simulink model "local_sequencer_harness1"  (R2018b)
settings: Solver=FixedStepDiscrete  StartTime=0  StopTime=8  FixedStep=1  RelTol=1e-3
undefined symbols (not defined in the file or in its folder): eof, sigbuilder_block, sldvsubsys, StateFlowModeType
libraries: sldvlib x21, simulink x6, hdlsllib x4
(part 2 of 2)

== stateflow chart local_sequencer_harness1/Test Unit (copied from local_sequencer)/Local Sequencer Subsystem/StateFlow ==
  settings: stateMachineType=MOORE_MACHINE  initializeOutput=1
  note: Make trigger and enable to chart?
  state INIT
    task_done = false;
    task_error = false;
    write = false;
    load_counter = false;
    ctrl = false;
    abort = false;
    increment = false;
    latch_inst_start = false;
    latch_addr = false;
    latch_function = false;
    reset = true;
  state FB_SELECT
    state LOAD_INST_START
      task_done = false;
      task_error = false;
      write = false;
      ctrl = false;
      abort = false;
      load_counter = true;
      increment = false;
      latch_inst_start = false;
      latch_addr = false;
      latch_function = false;
      reset = false;
    state LATCH_INST_START
      task_done = false;
      task_error = false;
      write = false;
      ctrl = false;
      abort = false;
      load_counter = false;
      increment = false;
      latch_inst_start = true;
      latch_addr = false;
      latch_function = true;
      reset = false;
    state INCREMENT_INST
      task_done = false;
      task_error = false;
      write = false;
      ctrl = false;
      abort = false;
      load_counter = false;
      increment = true;
      latch_inst_start = false;
      latch_addr = false;
      latch_function = false;
      reset = false;
    state INST_WAIT
      task_done = false;
      task_error = false;
      write = false;
      ctrl = false;
      abort = false;
      load_counter = false;
      increment = false;
      latch_inst_start = false;
      latch_addr = false;
      latch_function = false;
      reset = false;
    (default) -> LOAD_INST_START [order 1] : [recoverable]
    (default) -> LATCH_INST_START [order 2]
    LATCH_INST_START -> (junction 371)
    LOAD_INST_START -> (junction 371)
    (junction 371) -> FB_SELECT.INCREMENT_INST
    FB_SELECT.INCREMENT_INST -> FB_SELECT.INST_WAIT
  state FETCH
    state CTRL_LO
      task_done = false;
      task_error = false;
      write = false;
      ctrl = false;
      abort = false;
      load_counter = false;
      increment = false;
      latch_inst_start = false;
      latch_addr = false;
      latch_function = false;
      reset = false;
    state INCREMENT_INST
      task_done = false;
      task_error = false;
      write = false;
      ctrl = false;
      abort = false;
      load_counter = false;
      increment = true;
      latch_inst_start = false;
      latch_addr = false;
      latch_function = false;
      reset = false;
    state CTRL_HI
      task_done = false;
      task_error = false;
      write = false;
      ctrl = true;
      abort = false;
      load_counter = false;
      increment = false;
      latch_inst_start = false;
      latch_addr = false;
      latch_function = false;
      reset = false;
    state INST_WAIT
      task_done = false;
      task_error = false;
      write = false;
      ctrl = false;
      abort = false;
      load_counter = false;
      increment = false;
      latch_inst_start = false;
      latch_addr = false;
      latch_function = false;
      reset = false;
    state LATCH_ADDR
      task_done = false;
      task_error = false;
      write = false;
      ctrl = false;
      abort = false;
      load_counter = false;
      increment = false;
      latch_inst_start = false;
      latch_addr = true;
      latch_function = false;
      reset = false;
    state MEM_WAIT
      task_done = false;
      task_error = false;
      write = false;
      ctrl = false;
      abort = false;
      load_counter = false;
      increment = false;
      latch_inst_start = false;
      latch_addr = false;
      latch_function = false;
      reset = false;
    (default) -> FETCH.LATCH_ADDR
    FETCH.CTRL_LO -> FETCH.INCREMENT_INST
    FETCH.CTRL_HI -> FETCH.CTRL_LO
    FETCH.LATCH_ADDR -> MEM_WAIT
    MEM_WAIT -> FETCH.CTRL_HI
    FETCH.INCREMENT_INST -> FETCH.INST_WAIT
  state FB_EXECUTE
    state CTRL_HI
      task_done = false;
      task_error = false;
      write = false;
      ctrl = true;
      abort = false;
      load_counter = false;
      increment = false;
      latch_inst_start = false;
      latch_addr = false;
      latch_function = false;
      reset = false;
    state CTRL_LO
      task_done = false;
      task_error = false;
      write = false;
      ctrl = false;
      abort = false;
      load_counter = false;
      increment = false;
      latch_inst_start = false;
      latch_addr = false;
      latch_function = false;
      reset = false;
    (default) -> FB_EXECUTE.CTRL_HI
    FB_EXECUTE.CTRL_HI -> FB_EXECUTE.CTRL_LO
  state ERROR_STATE
    state CTRL_HI
      %set control and clear init
      task_done = false;
      task_error = false;
      write = false;
      ctrl = true;
      abort = false;
      load_counter = false;
      increment = false;
      latch_inst_start = false;
      latch_addr = false;
      latch_function = false;
      reset = false;
    state ABORT_CTRL_LO
      %task_error and init
      %unchanged
      task_done = false;
      task_error = task_error;
      write = false;
      ctrl = false;
      abort = false;
      load_counter = false;
      increment = false;
      latch_inst_start = false;
      latch_addr = false;
      latch_function = false;
      reset = false;
    state ABORT_CTRL_HI
      %set control, abort, and init
      task_done = false;
      task_error = true;
      write = false;
      ctrl = true;
      abort = true;
      load_counter = false;
      increment = false;
      latch_inst_start = false;
      latch_addr = false;
      latch_function = false;
      reset = false;
    (default) -> ERROR_STATE.CTRL_HI [order 1] : [recoverable]
    ERROR_STATE.CTRL_HI -> (junction 308)
    (default) -> ABORT_CTRL_HI [order 2]
    (junction 308) -> ABORT_CTRL_LO
    ABORT_CTRL_HI -> (junction 308)
  state WRITE
    state WRITE
      task_done = false;
      task_error = false;
      write = true;
      ctrl = false;
      abort = false;
      load_counter = false;
      increment = false;
      latch_inst_start = false;
      latch_addr = false;
      latch_function = false;
      reset = false;
    state INCREMENT_INST
      task_done = false;
      task_error = false;
      write = false;
      ctrl = false;
      abort = false;
      load_counter = false;
      increment = true;
      latch_inst_start = false;
      latch_addr = false;
      latch_function = false;
      reset = false;
    state CTRL_LO
      task_done = false;
      task_error = false;
      write = false;
      ctrl = false;
      abort = false;
      load_counter = false;
      increment = false;
      latch_inst_start = false;
      latch_addr = false;
      latch_function = false;
      reset = false;
    state CTRL_HI
      task_done = false;
      task_error = false;
      write = false;
      ctrl = true;
      abort = false;
      load_counter = false;
      increment = false;
      latch_inst_start = false;
      latch_addr = false;
      latch_function = false;
      reset = false;
    state LATCH_ADDR
      %latch current address
      task_done = false;
      task_error = false;
      write = false;
      ctrl = false;
      abort = false;
      load_counter = false;
      increment = false;
      latch_inst_start = false;
      latch_addr = true;
      latch_function = false;
      reset = false;
    state INST_WAIT
      task_done = false;
      task_error = false;
      write = false;
      ctrl = false;
      abort = false;
      load_counter = false;
      increment = false;
      latch_inst_start = false;
      latch_addr = false;
      latch_function = false;
      reset = false;
    (default) -> WRITE.LATCH_ADDR
    WRITE.LATCH_ADDR -> WRITE.CTRL_HI
    WRITE.CTRL_HI -> WRITE.CTRL_LO
    WRITE.WRITE -> WRITE.INCREMENT_INST
    WRITE.CTRL_LO -> WRITE.WRITE
    WRITE.INCREMENT_INST -> WRITE.INST_WAIT
  state FB_DONE
    state CTRL_HI
      task_done = false;
      task_error = false;
      write = false;
      ctrl = true;
      abort = false;
      load_counter = false;
      increment = false;
      latch_inst_start = false;
      latch_addr = false;
      latch_function = false;
      reset = false;
    state CTRL_LO
      task_done = false;
      task_error = false;
      write = false;
      ctrl = false;
      abort = false;
      load_counter = false;
      increment = false;
      latch_inst_start = false;
      latch_addr = false;
      latch_function = false;
      reset = false;
    (default) -> FB_DONE.CTRL_HI
    FB_DONE.CTRL_HI -> FB_DONE.CTRL_LO
  state TASK_DONE
    %signal task done
    task_done = true;
    task_error = false;
    write = false;
    ctrl = false;
    abort = false;
    load_counter = false;
    increment = false;
    latch_inst_start = false;
    latch_addr = false;
    latch_function = false;
    reset = false;
  FB_SELECT.INST_WAIT -> FETCH
  WRITE.INST_WAIT -> (junction 207)
  FB_DONE.CTRL_LO -> (junction 315) : [new_state]
  FB_EXECUTE.CTRL_LO -> WRITE : [new_state]
  FETCH.INST_WAIT -> (junction 204)
  ABORT_CTRL_LO -> (junction 220)
  (default) -> INIT
  (junction 220) -> INIT [order 2] : [~trigger]
  TASK_DONE -> INIT : [~trigger]
  INIT -> FB_SELECT : [trigger]
  (junction 220) -> FB_SELECT [order 1] : [recoverable]
  (junction 315) -> FB_SELECT [order 2]
  FETCH -> (junction 197)
  (junction 204) -> FETCH [order 2] : [state_iteration]
  (junction 204) -> FB_EXECUTE [order 1] : [new_state]
  FB_EXECUTE -> (junction 197)
  (junction 197) -> ERROR_STATE : [error]
  WRITE -> (junction 197)
  (junction 207) -> WRITE [order 2] : [state_iteration]
  (junction 207) -> FB_DONE [order 1] : [new_state]
  (junction 315) -> TASK_DONE [order 1] : [eof]
  data: task_done output boolean; task_error output boolean; write output boolean; ctrl output boolean; abort output boolean; load_counter output boolean; increment output boolean; latch_inst_start output boolean; latch_addr output boolean; latch_function output boolean; trigger input boolean; error input boolean; state_iteration input boolean; reset output boolean; new_state input boolean; recoverable input boolean; eof input boolean; StateFlowModeLS output Enum: StateFlowModeType

== matlab function local_sequencer_harness1/Test Unit (copied from local_sequencer)/Local Sequencer Subsystem/MATLAB Function ==
  data: code input; y output
function y = recoverable(code)
%#codegen

if(code)
    y = true;
else
    y = false;
end
